simulink model "m_rotor_v3"  (R2020b)
settings: Solver=VariableStepAuto  StartTime=0.0  StopTime=1  RelTol=1e-3
values from neighbouring files (symbols this model uses):
  Ator = pi*r^2    (= 0.00125663706144)    [INIT_rotor.m]
  bd = 20    [INIT_rotor.m]
  deltam = 3e-5    (= 3e-05)    [INIT_rotor.m]
  h0 = 100e-6    (= 0.0001)    [INIT_rotor.m]
  kd = 8e3    (= 8000)    [INIT_rotor.m]
  n = -3e+3    (= -3000)    [INIT_rotor.m]
  p0 = 1.08e5    (= 108000)    [INIT_rotor.m]
  p00 = 1.05e5    (= 105000)    [INIT_rotor.m]
  p1 = 1.08e5    (= 108000)    [INIT_rotor.m]
  p10 = 1.00e5    (= 100000)    [INIT_rotor.m]
  X10 = 1    [INIT_rotor.m]
  X20 = 0    [INIT_rotor.m]
  X30 = 200    [INIT_rotor.m]
undefined symbols (not defined in the file or in its folder): smiData, X, Y, Z
libraries: neural x80, sm_lib x21, nesl_utility x14, simulink x2, pid_lib x1
(part 4 of 4)

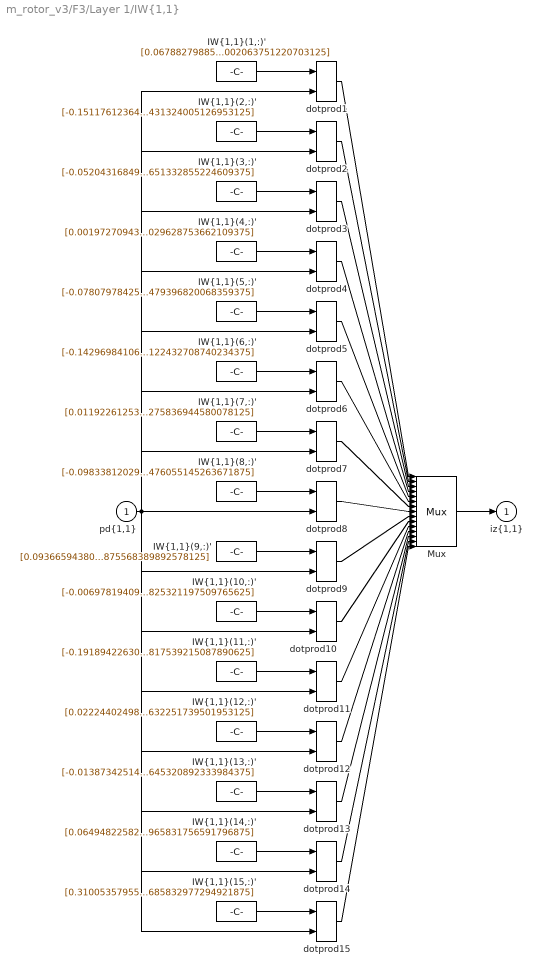
== system m_rotor_v3/F3/Layer 1/IW{1,1} ==
  "pd{1,1}" : Inport  PortDimensions=8
      mask Display: e = 0.06;c1 = [120 230 180]/255;c2 = ([120 230 180]+0)/(256+128);c3 = ([120 230 180]+128)/(256+128);patch([0 1 1 0],[0 0 1 1],c1);patch([0 1 1 1-e 1-e 0+e],[0 0 1 1-e 0+e 0+e],c2);patch([0 0 1 1-e 0+e 0+e],[0 1 1 1-e 1-e 0+e],c3);plot([0 1 1 0 0],[0 0 1 1 0]);
  "IW{1,1}(1,:)'" : Constant  Value=[0.06788279885655380818665349806906306184828281402587890625;-0.00992236614156143115206276661410811357200145721435546875;0.128807470069277008040131704547093249857425689697265625;-2.07557374820626261424649783293716609477996826171875;-1.3371842639701483346215127312461845576763153076171875;-2.173773926338138817726530760410241782665252685546875;-0.854299781709458638800924745737574994564056396484375;0.06477886523293803489043085619414341636002063751220703125]
      mask Display: e = 0.06;c1 = [120 150 230]/255;c2 = ([120 150 230]+0)/383;c3 = ([120 150 230]+128)/383;patch([0 1 1 0],[0 0 1 1],c1);patch([0 1 1 1-e 1-e 0+e],[0 0 1 1-e 0+e 0+e],c2);patch([0 0 1 1-e 0+e 0+e],[0 1 1 1-e 1-e 0+e],c3);plot([0 1 1 0 0],[0 0 1 1 0]);disp('Weights');
  "IW{1,1}(10,:)'" : Constant  Value=[-0.006978194095090421711358175116401980631053447723388671875;0.00922221332153015660448858170639141462743282318115234375;-0.330894108761513872085657794741564430296421051025390625;0.8886342899794936744939377604168839752674102783203125;-0.351152275670796931716921562838251702487468719482421875;0.9474812931835525642298989623668603599071502685546875;1.021305796765827000882609354448504745960235595703125;-0.037725419671657024756061815651264623738825321197509765625]
      mask Display: e = 0.06;c1 = [120 150 230]/255;c2 = ([120 150 230]+0)/383;c3 = ([120 150 230]+128)/383;patch([0 1 1 0],[0 0 1 1],c1);patch([0 1 1 1-e 1-e 0+e],[0 0 1 1-e 0+e 0+e],c2);patch([0 0 1 1-e 0+e 0+e],[0 1 1 1-e 1-e 0+e],c3);plot([0 1 1 0 0],[0 0 1 1 0]);disp('Weights');
  "IW{1,1}(11,:)'" : Constant  Value=[-0.1918942263094554900870747360386303626000881195068359375;-0.0045254450572274999842203868638534913770854473114013671875;0.898112362451640944271957778255455195903778076171875;0.216610886716492812009704493902972899377346038818359375;-0.5903638625466645084571837287512607872486114501953125;-2.03988383709788489994707560981623828411102294921875;0.133448489177298179608754935543402098119258880615234375;0.149400957588209204462970092208706773817539215087890625]
      mask Display: e = 0.06;c1 = [120 150 230]/255;c2 = ([120 150 230]+0)/383;c3 = ([120 150 230]+128)/383;patch([0 1 1 0],[0 0 1 1],c1);patch([0 1 1 1-e 1-e 0+e],[0 0 1 1-e 0+e 0+e],c2);patch([0 0 1 1-e 0+e 0+e],[0 1 1 1-e 1-e 0+e],c3);plot([0 1 1 0 0],[0 0 1 1 0]);disp('Weights');
  "IW{1,1}(12,:)'" : Constant  Value=[0.0222440249845849737087011277480996795929968357086181640625;0.00650835675493242372946500751140774809755384922027587890625;0.2126146796901738633689404878168716095387935638427734375;0.22473885325326126150002892245538532733917236328125;-0.77026826774832157784800301669747568666934967041015625;-0.42125467116819759194612515784683637320995330810546875;0.83276323841456501018143399051041342318058013916015625;0.017557852814675374564234999752443400211632251739501953125]
      mask Display: e = 0.06;c1 = [120 150 230]/255;c2 = ([120 150 230]+0)/383;c3 = ([120 150 230]+128)/383;patch([0 1 1 0],[0 0 1 1],c1);patch([0 1 1 1-e 1-e 0+e],[0 0 1 1-e 0+e 0+e],c2);patch([0 0 1 1-e 0+e 0+e],[0 1 1 1-e 1-e 0+e],c3);plot([0 1 1 0 0],[0 0 1 1 0]);disp('Weights');
  "IW{1,1}(13,:)'" : Constant  Value=[-0.01387342514656162047181897634118286077864468097686767578125;0.01297421504082907350863251849659718573093414306640625;-0.631599189159698592987979282042942941188812255859375;-0.9796428852581460233750476618297398090362548828125;-0.0383016700428938372535725420675589703023433685302734375;-1.6157790195434416080644268731703050434589385986328125;-1.0822132089536109500471638966700993478298187255859375;0.052192302752546236577213534246766357682645320892333984375]
      mask Display: e = 0.06;c1 = [120 150 230]/255;c2 = ([120 150 230]+0)/383;c3 = ([120 150 230]+128)/383;patch([0 1 1 0],[0 0 1 1],c1);patch([0 1 1 1-e 1-e 0+e],[0 0 1 1-e 0+e 0+e],c2);patch([0 0 1 1-e 0+e 0+e],[0 1 1 1-e 1-e 0+e],c3);plot([0 1 1 0 0],[0 0 1 1 0]);disp('Weights');
  "IW{1,1}(14,:)'" : Constant  Value=[0.06494822582515873132802397549312445335090160369873046875;0.01179147852846387616032597378534774179570376873016357421875;-0.55416769562306011920327364350669085979461669921875;-0.7851185296991458617554826560080982744693756103515625;-0.353385480256569295409718733935733325779438018798828125;1.9326126031133357141555961788981221616268157958984375;0.318004305208750615019397400828893296420574188232421875;-0.041408834171954171654572718352937954477965831756591796875]
      mask Display: e = 0.06;c1 = [120 150 230]/255;c2 = ([120 150 230]+0)/383;c3 = ([120 150 230]+128)/383;patch([0 1 1 0],[0 0 1 1],c1);patch([0 1 1 1-e 1-e 0+e],[0 0 1 1-e 0+e 0+e],c2);patch([0 0 1 1-e 0+e 0+e],[0 1 1 1-e 1-e 0+e],c3);plot([0 1 1 0 0],[0 0 1 1 0]);disp('Weights');
  "IW{1,1}(15,:)'" : Constant  Value=[0.310053579551866909103097214028821326792240142822265625;-0.003967058471211982496884562721106703975237905979156494140625;-1.1384331891469832154228924991912208497524261474609375;-0.1774212528405465227887560786257381550967693328857421875;1.0456562539913416554071545760962180793285369873046875;2.177732673321708833924503778689540922641754150390625;-0.436451307036899549540720499862800352275371551513671875;-0.2422999450589031489311508948958362452685832977294921875]
      mask Display: e = 0.06;c1 = [120 150 230]/255;c2 = ([120 150 230]+0)/383;c3 = ([120 150 230]+128)/383;patch([0 1 1 0],[0 0 1 1],c1);patch([0 1 1 1-e 1-e 0+e],[0 0 1 1-e 0+e 0+e],c2);patch([0 0 1 1-e 0+e 0+e],[0 1 1 1-e 1-e 0+e],c3);plot([0 1 1 0 0],[0 0 1 1 0]);disp('Weights');
  "IW{1,1}(2,:)'" : Constant  Value=[-0.1511761236496747262680884205110487528145313262939453125;-0.00881789659697155940587531830487932893447577953338623046875;-0.1261543085943037656448950656340457499027252197265625;0.489396239657587217575240856604068540036678314208984375;-0.2207616966116522638774455344901070930063724517822265625;0.251424731887772423544191724431584589183330535888671875;0.097557007687249230887260864619747735559940338134765625;0.0239275744022753762696442692003984120674431324005126953125]
      mask Display: e = 0.06;c1 = [120 150 230]/255;c2 = ([120 150 230]+0)/383;c3 = ([120 150 230]+128)/383;patch([0 1 1 0],[0 0 1 1],c1);patch([0 1 1 1-e 1-e 0+e],[0 0 1 1-e 0+e 0+e],c2);patch([0 0 1 1-e 0+e 0+e],[0 1 1 1-e 1-e 0+e],c3);plot([0 1 1 0 0],[0 0 1 1 0]);disp('Weights');
  "IW{1,1}(3,:)'" : Constant  Value=[-0.05204316849955237245239914045669138431549072265625;0.00142568734179253863401937163501997929415665566921234130859375;-1.860726472222154814772920872201211750507354736328125;-1.3699586386795095105384234557277522981166839599609375;-0.288754708460629838651101408686372451484203338623046875;0.43689781072489697333338654061662964522838592529296875;-1.3054144450678315525493644599919207394123077392578125;0.005906429554605130416433667051023803651332855224609375]
      mask Display: e = 0.06;c1 = [120 150 230]/255;c2 = ([120 150 230]+0)/383;c3 = ([120 150 230]+128)/383;patch([0 1 1 0],[0 0 1 1],c1);patch([0 1 1 1-e 1-e 0+e],[0 0 1 1-e 0+e 0+e],c2);patch([0 0 1 1-e 0+e 0+e],[0 1 1 1-e 1-e 0+e],c3);plot([0 1 1 0 0],[0 0 1 1 0]);disp('Weights');
  "IW{1,1}(4,:)'" : Constant  Value=[0.001972709436021187479060046143786166794598102569580078125;-0.007549715445535030988732927426099195145070552825927734375;-1.196959391696092556145458729588426649570465087890625;-0.65884191472665321054336118322680704295635223388671875;-0.1867951756140261154737203241893439553678035736083984375;0.431106399485792712855669606142328120768070220947265625;-0.581805685047673382115362983313389122486114501953125;0.056432614527383816172001473887576139532029628753662109375]
      mask Display: e = 0.06;c1 = [120 150 230]/255;c2 = ([120 150 230]+0)/383;c3 = ([120 150 230]+128)/383;patch([0 1 1 0],[0 0 1 1],c1);patch([0 1 1 1-e 1-e 0+e],[0 0 1 1-e 0+e 0+e],c2);patch([0 0 1 1-e 0+e 0+e],[0 1 1 1-e 1-e 0+e],c3);plot([0 1 1 0 0],[0 0 1 1 0]);disp('Weights');
  "IW{1,1}(5,:)'" : Constant  Value=[-0.07807978425676752320949702834695926867425441741943359375;-0.00677429953288709828240765631335307261906564235687255859375;-0.0664314126019382999999152161763049662113189697265625;-0.386955493755659352128617456401116214692592620849609375;-0.0960269927478801521569806709521799348294734954833984375;-0.01720314009759908724372934329949202947318553924560546875;0.057611214507576093135643446885296725668013095855712890625;-0.0248487489313878005814384408722617081366479396820068359375]
      mask Display: e = 0.06;c1 = [120 150 230]/255;c2 = ([120 150 230]+0)/383;c3 = ([120 150 230]+128)/383;patch([0 1 1 0],[0 0 1 1],c1);patch([0 1 1 1-e 1-e 0+e],[0 0 1 1-e 0+e 0+e],c2);patch([0 0 1 1-e 0+e 0+e],[0 1 1 1-e 1-e 0+e],c3);plot([0 1 1 0 0],[0 0 1 1 0]);disp('Weights');
  "IW{1,1}(6,:)'" : Constant  Value=[-0.1429698410676345232683814856500248424708843231201171875;0.06679343247472328826130905099489609710872173309326171875;0.78610319187799693185780824933317489922046661376953125;0.98970498789565641839516274558263830840587615966796875;0.85264808828135041363083246324094943702220916748046875;-1.9128706056098938592668901037541218101978302001953125;0.838971287901387086094473488628864288330078125;0.1026202929340290503912314079570933245122432708740234375]
      mask Display: e = 0.06;c1 = [120 150 230]/255;c2 = ([120 150 230]+0)/383;c3 = ([120 150 230]+128)/383;patch([0 1 1 0],[0 0 1 1],c1);patch([0 1 1 1-e 1-e 0+e],[0 0 1 1-e 0+e 0+e],c2);patch([0 0 1 1-e 0+e 0+e],[0 1 1 1-e 1-e 0+e],c3);plot([0 1 1 0 0],[0 0 1 1 0]);disp('Weights');
  "IW{1,1}(7,:)'" : Constant  Value=[0.01192261253205783265440853568861712119542062282562255859375;0.002953547315193994111937048074878475745208561420440673828125;0.80887583328624590439659414187190122902393341064453125;-0.1311186120981299441101697311751195229589939117431640625;0.1442848684722133623115070122366887517273426055908203125;-0.25060501965799419910041478942730464041233062744140625;0.407150347884929264541398197252419777214527130126953125;-0.08340267370550531744743949502662871964275836944580078125]
      mask Display: e = 0.06;c1 = [120 150 230]/255;c2 = ([120 150 230]+0)/383;c3 = ([120 150 230]+128)/383;patch([0 1 1 0],[0 0 1 1],c1);patch([0 1 1 1-e 1-e 0+e],[0 0 1 1-e 0+e 0+e],c2);patch([0 0 1 1-e 0+e 0+e],[0 1 1 1-e 1-e 0+e],c3);plot([0 1 1 0 0],[0 0 1 1 0]);disp('Weights');
  "IW{1,1}(8,:)'" : Constant  Value=[-0.0983381202998495351774721484616748057305812835693359375;-0.002896860992941151409507671843357456964440643787384033203125;0.1773862169213134831746714326072833500802516937255859375;0.7067698616238973219338959097512997686862945556640625;-0.239147493231804675328788789556710980832576751708984375;0.1555922986075080338697063098152284510433673858642578125;0.52311960761349907134132308783591724932193756103515625;0.0264900577877667901816050033403371344320476055145263671875]
      mask Display: e = 0.06;c1 = [120 150 230]/255;c2 = ([120 150 230]+0)/383;c3 = ([120 150 230]+128)/383;patch([0 1 1 0],[0 0 1 1],c1);patch([0 1 1 1-e 1-e 0+e],[0 0 1 1-e 0+e 0+e],c2);patch([0 0 1 1-e 0+e 0+e],[0 1 1 1-e 1-e 0+e],c3);plot([0 1 1 0 0],[0 0 1 1 0]);disp('Weights');
  "IW{1,1}(9,:)'" : Constant  Value=[0.09366594380494457083852211098928819410502910614013671875;-0.01440292874345421199333561190769614768214523792266845703125;-0.3520744791741849955002408023574389517307281494140625;-0.8998918382846816665932010437245480716228485107421875;0.374977485732819026953421825965051539242267608642578125;-0.131297970009684183967380022295401431620121002197265625;-0.957166522100834527009283192455768585205078125;-0.0689537204583486051934215765868430025875568389892578125]
      mask Display: e = 0.06;c1 = [120 150 230]/255;c2 = ([120 150 230]+0)/383;c3 = ([120 150 230]+128)/383;patch([0 1 1 0],[0 0 1 1],c1);patch([0 1 1 1-e 1-e 0+e],[0 0 1 1-e 0+e 0+e],c2);patch([0 0 1 1-e 0+e 0+e],[0 1 1 1-e 1-e 0+e],c3);plot([0 1 1 0 0],[0 0 1 1 0]);disp('Weights');
  Mux : Mux  Inputs=15
      mask Display: e = 0.06;c1 = [120 150 230]/255;c2 = ([120 150 230]+0)/383;c3 = ([120 150 230]+128)/383;patch([0 1 1 0],[0 0 1 1],c1);patch([0 1 1 1-e 1-e 0+e],[0 0 1 1-e 0+e 0+e],c2);patch([0 0 1 1-e 0+e 0+e],[0 1 1 1-e 1-e 0+e],c3);plot([0 1 1 0 0],[0 0 1 1 0]);disp('Mux');
  dotprod{1..15} (15 alike) : neural/Weight Functions/dotprod
  "iz{1,1}" : Outport
      mask Display: e = 0.06;c1 = [120 230 180]/255;c2 = ([120 230 180]+0)/(256+128);c3 = ([120 230 180]+128)/(256+128);patch([0 1 1 0],[0 0 1 1],c1);patch([0 1 1 1-e 1-e 0+e],[0 0 1 1-e 0+e 0+e],c2);patch([0 0 1 1-e 0+e 0+e],[0 1 1 1-e 1-e 0+e],c3);plot([0 1 1 0 0],[0 0 1 1 0]);
  wires:
  "IW{1,1}(1,:)'"/1 -> dotprod1/1
  "pd{1,1}"/1 -> dotprod1/2, dotprod2/2, dotprod3/2, dotprod4/2, dotprod5/2, dotprod6/2, dotprod7/2, dotprod8/2, dotprod9/2, dotprod10/2, dotprod11/2, dotprod12/2, dotprod13/2, dotprod14/2, dotprod15/2
  dotprod1/1 -> Mux/1
  "IW{1,1}(2,:)'"/1 -> dotprod2/1
  dotprod2/1 -> Mux/2
  "IW{1,1}(3,:)'"/1 -> dotprod3/1
  dotprod3/1 -> Mux/3
  "IW{1,1}(4,:)'"/1 -> dotprod4/1
  dotprod4/1 -> Mux/4
  "IW{1,1}(5,:)'"/1 -> dotprod5/1
  dotprod5/1 -> Mux/5
  "IW{1,1}(6,:)'"/1 -> dotprod6/1
  dotprod6/1 -> Mux/6
  "IW{1,1}(7,:)'"/1 -> dotprod7/1
  dotprod7/1 -> Mux/7
  "IW{1,1}(8,:)'"/1 -> dotprod8/1
  dotprod8/1 -> Mux/8
  "IW{1,1}(9,:)'"/1 -> dotprod9/1
  dotprod9/1 -> Mux/9
  "IW{1,1}(10,:)'"/1 -> dotprod10/1
  dotprod10/1 -> Mux/10
  "IW{1,1}(11,:)'"/1 -> dotprod11/1
  dotprod11/1 -> Mux/11
  "IW{1,1}(12,:)'"/1 -> dotprod12/1
  dotprod12/1 -> Mux/12
  "IW{1,1}(13,:)'"/1 -> dotprod13/1
  dotprod13/1 -> Mux/13
  "IW{1,1}(14,:)'"/1 -> dotprod14/1
  dotprod14/1 -> Mux/14
  "IW{1,1}(15,:)'"/1 -> dotprod15/1
  dotprod15/1 -> Mux/15
  Mux/1 -> "iz{1,1}"/1

== system m_rotor_v3/F3/Layer 2/Delays 1 ==
  "p{2}" : Inport  PortDimensions=15
      mask Display: e = 0.06;c1 = [120 230 180]/255;c2 = ([120 230 180]+0)/(256+128);c3 = ([120 230 180]+128)/(256+128);patch([0 1 1 0],[0 0 1 1],c1);patch([0 1 1 1-e 1-e 0+e],[0 0 1 1-e 0+e 0+e],c2);patch([0 0 1 1-e 0+e 0+e],[0 1 1 1-e 1-e 0+e],c3);plot([0 1 1 0 0],[0 0 1 1 0]);
  mux : Mux  Inputs=1
      mask Display: e = 0.06;c1 = [120 150 230]/255;c2 = ([120 150 230]+0)/383;c3 = ([120 150 230]+128)/383;patch([0 1 1 0],[0 0 1 1],c1);patch([0 1 1 1-e 1-e 0+e],[0 0 1 1-e 0+e 0+e],c2);patch([0 0 1 1-e 0+e 0+e],[0 1 1 1-e 1-e 0+e],c3);plot([0 1 1 0 0],[0 0 1 1 0]);disp('Mux')
  "pd{2,1}" : Outport
      mask Display: e = 0.06;c1 = [120 230 180]/255;c2 = ([120 230 180]+0)/(256+128);c3 = ([120 230 180]+128)/(256+128);patch([0 1 1 0],[0 0 1 1],c1);patch([0 1 1 1-e 1-e 0+e],[0 0 1 1-e 0+e 0+e],c2);patch([0 0 1 1-e 0+e 0+e],[0 1 1 1-e 1-e 0+e],c3);plot([0 1 1 0 0],[0 0 1 1 0]);
  wires:
  "p{2}"/1 -> mux/1
  mux/1 -> "pd{2,1}"/1

== system m_rotor_v3/F3/Layer 2/LW{2,1} ==
  "ad{2,1}" : Inport  PortDimensions=15
      mask Display: e = 0.06;c1 = [120 230 180]/255;c2 = ([120 230 180]+0)/(256+128);c3 = ([120 230 180]+128)/(256+128);patch([0 1 1 0],[0 0 1 1],c1);patch([0 1 1 1-e 1-e 0+e],[0 0 1 1-e 0+e 0+e],c2);patch([0 0 1 1-e 0+e 0+e],[0 1 1 1-e 1-e 0+e],c3);plot([0 1 1 0 0],[0 0 1 1 0]);
  "IW{2,1}(1,:)'" : Constant  Value=[-3.617594306433918216470146944629959762096405029296875;4.02640558418821559172329216380603611469268798828125;-3.234515089768903006728351101628504693508148193359375;-1.4739495354445899533146757676149718463420867919921875;2.8710019130520691987840109504759311676025390625;0.1363723444796345052321129287520307116210460662841796875;-1.496996753744781916140027533401735126972198486328125;-4.67582619968248192066084811813198029994964599609375;-1.2046706811599718900396283061127178370952606201171875;-4.35845704992661797660957745392806828022003173828125;-2.28128825068953222654499768395908176898956298828125;5.3857038849677110192715190351009368896484375;2.5065702664579792013910264358855783939361572265625;-2.23875268234986268822694910340942442417144775390625;-1.1284468873998025895133423546212725341320037841796875]
      mask Display: e = 0.06;c1 = [120 150 230]/255;c2 = ([120 150 230]+0)/383;c3 = ([120 150 230]+128)/383;patch([0 1 1 0],[0 0 1 1],c1);patch([0 1 1 1-e 1-e 0+e],[0 0 1 1-e 0+e 0+e],c2);patch([0 0 1 1-e 0+e 0+e],[0 1 1 1-e 1-e 0+e],c3);plot([0 1 1 0 0],[0 0 1 1 0]);disp('weights');
  Mux : Mux  Inputs=1
      mask Display: e = 0.06;c1 = [120 150 230]/255;c2 = ([120 150 230]+0)/383;c3 = ([120 150 230]+128)/383;patch([0 1 1 0],[0 0 1 1],c1);patch([0 1 1 1-e 1-e 0+e],[0 0 1 1-e 0+e 0+e],c2);patch([0 0 1 1-e 0+e 0+e],[0 1 1 1-e 1-e 0+e],c3);plot([0 1 1 0 0],[0 0 1 1 0]);disp('Mux');
  dotprod1 : neural/Weight Functions/dotprod
  "lz{2,1}" : Outport
      mask Display: e = 0.06;c1 = [120 230 180]/255;c2 = ([120 230 180]+0)/(256+128);c3 = ([120 230 180]+128)/(256+128);patch([0 1 1 0],[0 0 1 1],c1);patch([0 1 1 1-e 1-e 0+e],[0 0 1 1-e 0+e 0+e],c2);patch([0 0 1 1-e 0+e 0+e],[0 1 1 1-e 1-e 0+e],c3);plot([0 1 1 0 0],[0 0 1 1 0]);
  wires:
  "IW{2,1}(1,:)'"/1 -> dotprod1/1
  "ad{2,1}"/1 -> dotprod1/2
  dotprod1/1 -> Mux/1
  Mux/1 -> "lz{2,1}"/1
